simulink model "NowWereHere2018"  (R2018b)
settings: Solver=VariableStepAuto  StartTime=0.0  StopTime=120  MaxStep=10e-3  RelTol=1e-3
libraries: simulink x1, simulink_extras x1
settings Model: Creator=einarsu  LastModifiedBy=krist
settings OptimizationCC: LifeSpan=inf
settings SFSimCC: SimUseLocalCustomCode=off
settings RTWCC: RTWUseLocalCustomCode=off
settings CodeAppCC: StateflowObjectComments=on

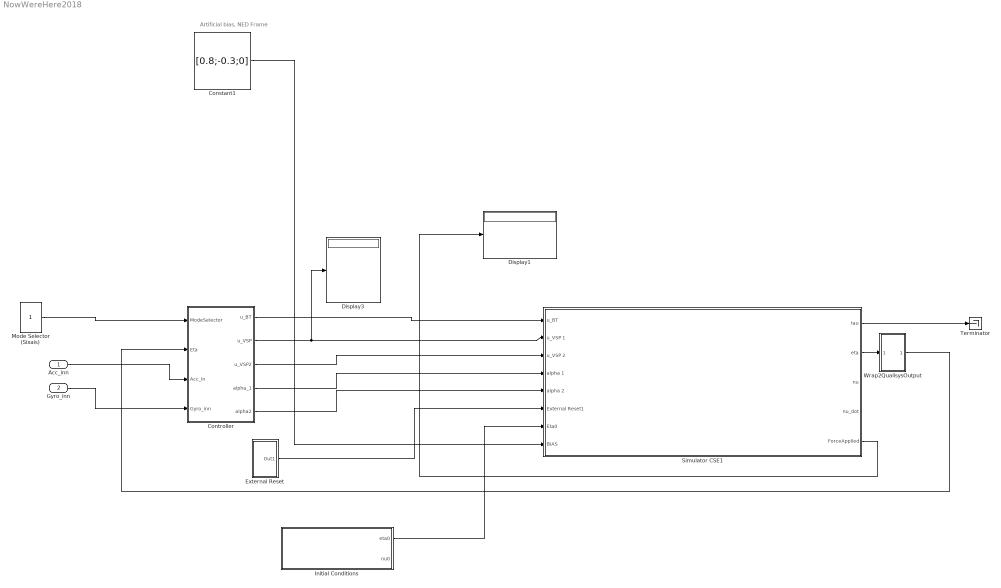
== system NowWereHere2018 ==
  note: Artificial bias, NED Frame
  Acc_inn : Inport
  Gyro_inn : Inport  Port=2
  Constant1 : Constant  Value=[0.8;-0.3;0]
  Controller : Subsystem
  Display1 : Display
  Display3 : Display
  External Reset : Subsystem
  "Initial Conditions " : Subsystem
  Mode Selector (Sixais) : Constant
  Simulator CSE1 : Subsystem
  Terminator : Terminator
  "Wrap2QualisysOutput " : Subsystem
  wires:
  Controller/1(u_BT) -> Simulator CSE1/1(u_BT)
  Controller/4(alpha_1) -> Simulator CSE1/4(alpha 1)
  Controller/2(u_VSP) -> Display3/1, Simulator CSE1/2(u_VSP 1)
  Controller/5(alpha2) -> Simulator CSE1/5(alpha 2)
  Controller/3("u_VSP2 ") -> Simulator CSE1/3(u_VSP 2)
  Simulator CSE1/1(tau) -> Terminator/1
  External Reset/1(Out1) -> Simulator CSE1/6(External Reset1)
  "Initial Conditions "/1(eta0) -> Simulator CSE1/7(Eta0)
  Mode Selector (Sixais)/1 -> Controller/1(ModeSelector)
  Simulator CSE1/2(eta) -> "Wrap2QualisysOutput "/1(In1)
  Acc_inn/1 -> Controller/3(Acc_in)
  Gyro_inn/1 -> Controller/4(Gyro_inn)
  Simulator CSE1/5(ForceApplied) -> Display1/1
  Constant1/1 -> Simulator CSE1/8(BIAS)
  "Wrap2QualisysOutput "/1(Out1) -> Controller/2(Eta)

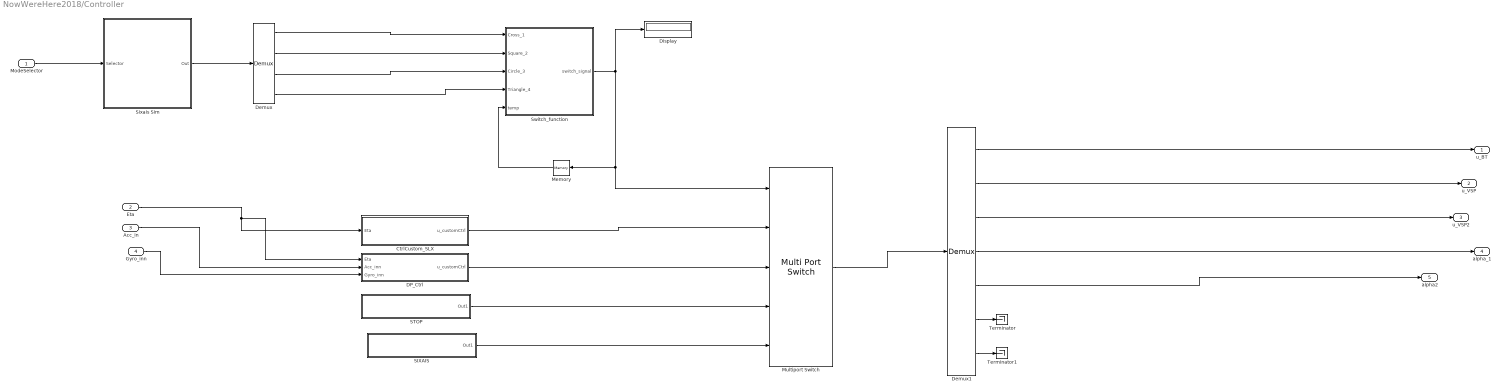
== system NowWereHere2018/Controller ==
  ModeSelector : Inport
  Eta : Inport  Port=2
  Acc_in : Inport  Port=3
  Gyro_inn : Inport  Port=4
  CtrlCustom_SLX : Subsystem
  DP_Ctrl : Subsystem
  Demux : Demux
  Demux1 : Demux  Outputs=7
  Display : Display
  Memory : Memory  InitialCondition=4
  Multiport Switch : MultiPortSwitch  Inputs=4
  SIXAIS : Subsystem
  STOP : Subsystem
  Sixais Sim : MATLAB Function  TreatAsAtomicUnit=on
  Switch_function : MATLAB Function  TreatAsAtomicUnit=on
  Terminator : Terminator
  Terminator1 : Terminator
  u_BT : Outport  VectorParamsAs1DForOutWhenUnconnected=off
  u_VSP : Outport  Port=2  VectorParamsAs1DForOutWhenUnconnected=off
  "u_VSP2 " : Outport  Port=3  VectorParamsAs1DForOutWhenUnconnected=off
  alpha_1 : Outport  Port=4  VectorParamsAs1DForOutWhenUnconnected=off
  alpha2 : Outport  Port=5  VectorParamsAs1DForOutWhenUnconnected=off
  wires:
  Switch_function/1(switch_signal) -> Memory/1, Multiport Switch/1, Display/1
  Memory/1 -> Switch_function/5(temp)
  CtrlCustom_SLX/1(u_customCtrl) -> Multiport Switch/2
  Demux/1 -> Switch_function/1(Cross_1)
  Demux/2 -> Switch_function/2(Square_2)
  Demux/3 -> Switch_function/3(Circle_3)
  Demux/4 -> Switch_function/4(Triangle_4)
  Sixais Sim/1(Out) -> Demux/1
  ModeSelector/1 -> Sixais Sim/1(Selector)
  DP_Ctrl/1(u_customCtrl) -> Multiport Switch/3
  STOP/1(Out1) -> Multiport Switch/4
  SIXAIS/1(Out1) -> Multiport Switch/5
  Eta/1 -> DP_Ctrl/1(Eta), CtrlCustom_SLX/1(Eta)
  Acc_in/1 -> DP_Ctrl/2(Acc_inn)
  Gyro_inn/1 -> DP_Ctrl/3(Gyro_inn)
  Multiport Switch/1 -> Demux1/1
  Demux1/1 -> u_BT/1
  Demux1/2 -> u_VSP/1
  Demux1/3 -> "u_VSP2 "/1
  Demux1/4 -> alpha_1/1
  Demux1/5 -> alpha2/1
  Demux1/6 -> Terminator/1
  Demux1/7 -> Terminator1/1

== system NowWereHere2018/External Reset ==
  note: Most relevant for Real-Time Simulations...
  Constant : Constant  Value=0
  Out1 : Outport  VectorParamsAs1DForOutWhenUnconnected=off
  wires:
  Constant/1 -> Out1/1

== system NowWereHere2018/Initial Conditions  ==
  Eta0 : Constant  Value=zeros(3,1)
  "V0 " : Constant  Value=zeros(3,1)
  eta0 : Outport  VectorParamsAs1DForOutWhenUnconnected=off
  nu0 : Outport  Port=2  VectorParamsAs1DForOutWhenUnconnected=off
  wires:
  "V0 "/1 -> nu0/1
  Eta0/1 -> eta0/1

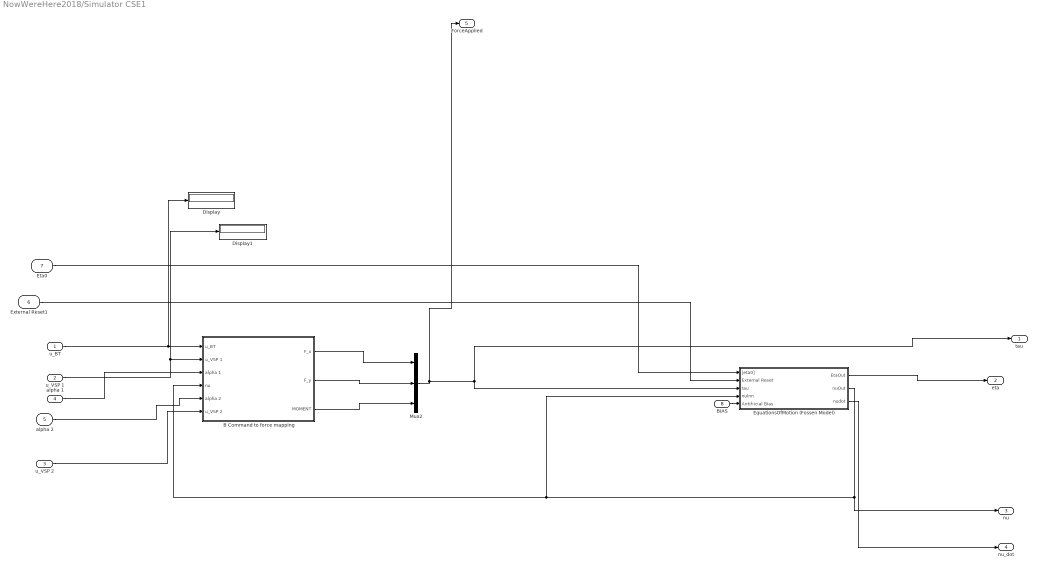
== system NowWereHere2018/Simulator CSE1 ==
  u_BT : Inport
  u_VSP 1 : Inport  Port=2
  u_VSP 2 : Inport  Port=3
  alpha 1 : Inport  Port=4
  alpha 2 : Inport  Port=5
  External Reset1 : Inport  Port=6
  Eta0 : Inport  Port=7
  BIAS : Inport  Port=8
  B Command to force mapping : Subsystem
  Display : Display
  Display1 : Display
  EquationsOfMotion (Fossen Model) : Subsystem
  Mux2 : Mux  Inputs=3
  tau : Outport  VectorParamsAs1DForOutWhenUnconnected=off
  eta : Outport  Port=2  VectorParamsAs1DForOutWhenUnconnected=off
  nu : Outport  Port=3  VectorParamsAs1DForOutWhenUnconnected=off
  nu_dot : Outport  Port=4  VectorParamsAs1DForOutWhenUnconnected=off
  ForceApplied : Outport  Port=5  VectorParamsAs1DForOutWhenUnconnected=off
  wires:
  alpha 2/1 -> B Command to force mapping/5(alpha 2)
  B Command to force mapping/2("F_y ") -> Mux2/2
  B Command to force mapping/1(F_x) -> Mux2/1
  u_VSP 1/1 -> B Command to force mapping/2(u_VSP 1), Display1/1
  alpha 1/1 -> B Command to force mapping/3(alpha 1)
  u_BT/1 -> B Command to force mapping/1(u_BT), Display/1
  u_VSP 2/1 -> B Command to force mapping/6(u_VSP 2)
  EquationsOfMotion (Fossen Model)/2(nuOut) -> B Command to force mapping/4(nu), EquationsOfMotion (Fossen Model)/4(nuInn), nu/1
  Eta0/1 -> EquationsOfMotion (Fossen Model)/1("[eta0] ")
  External Reset1/1 -> EquationsOfMotion (Fossen Model)/2(External Reset)
  Mux2/1 -> ForceApplied/1, EquationsOfMotion (Fossen Model)/3(tau), tau/1
  EquationsOfMotion (Fossen Model)/1(EtaOut) -> eta/1
  EquationsOfMotion (Fossen Model)/3(nudot) -> nu_dot/1
  B Command to force mapping/3("MOMENT ") -> Mux2/3
  BIAS/1 -> EquationsOfMotion (Fossen Model)/5(Aritifiicial BIas)

== system NowWereHere2018/Wrap2QualisysOutput  ==
  In1 : Inport
  Demux : Demux  Outputs=3
  Gain : Gain  Gain=1000
  Gain1 : Gain  Gain=1000
  Gain2 : Gain  Gain=180/pi
  Mux : Mux  Inputs=3
  Wrap2psi : MATLAB Function  TreatAsAtomicUnit=on
  Out1 : Outport  VectorParamsAs1DForOutWhenUnconnected=off
  wires:
  Mux/1 -> Out1/1
  In1/1 -> Demux/1
  Demux/3 -> Wrap2psi/1(u)
  Demux/1 -> Gain/1
  Demux/2 -> Gain1/1
  Gain/1 -> Mux/1
  Gain1/1 -> Mux/2
  Gain2/1 -> Mux/3
  Wrap2psi/1(yQualisus) -> Gain2/1

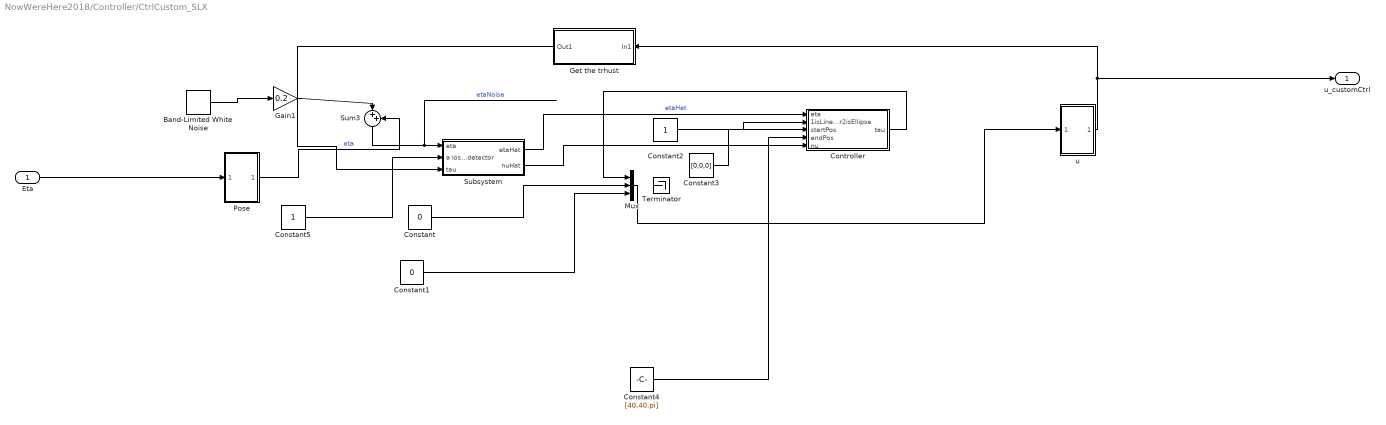
== system NowWereHere2018/Controller/CtrlCustom_SLX ==
  Eta : Inport
  Band-Limited White Noise : simulink/Sources/Band-Limited White Noise  Cov=[0.1]  Ts=0.1  seed=[23341]
  Constant : Constant  Value=0
  Constant1 : Constant  Value=0
  Constant2 : Constant
  Constant3 : Constant  Value=[0,0,0]
  Constant4 : Constant  Value=[40,40,pi]
  Constant5 : Constant
  Controller : Subsystem
  Gain1 : Gain  Gain=0.2
  Get the trhust : Subsystem
  Mux : Mux  Inputs=3
  Pose : Subsystem
  Subsystem : Subsystem
  Sum3 : Sum  Inputs=|++
  Terminator : Terminator
  u : Subsystem
  u_customCtrl : Outport  VectorParamsAs1DForOutWhenUnconnected=off
  wires:
  Eta/1 -> Pose/1(eta)
  Constant1/1 -> Mux/3
  Constant/1 -> Mux/2
  Pose/1(QTM) -> Sum3/2  "eta"
  Subsystem/1(etaHat) -> Controller/1(eta)  "etaHat"
  Constant5/1 -> Subsystem/2(a loss-of-signal detector)
  u/1(Out1) -> Get the trhust/1(In1), u_customCtrl/1
  Get the trhust/1(Out1) -> Subsystem/3(tau)
  Band-Limited White Noise/1 -> Gain1/1
  Gain1/1 -> Sum3/1
  Sum3/1 -> Subsystem/1(eta)  "etaNoise"
  Controller/1(tau) -> Mux/1
  Mux/1 -> u/1(In1)
  Constant2/1 -> Controller/2(1isLinear2isEllipse)
  Constant3/1 -> Controller/3(startPos)
  Constant4/1 -> Controller/4(endPos)
  Subsystem/2(nuHat) -> Controller/5(nu)

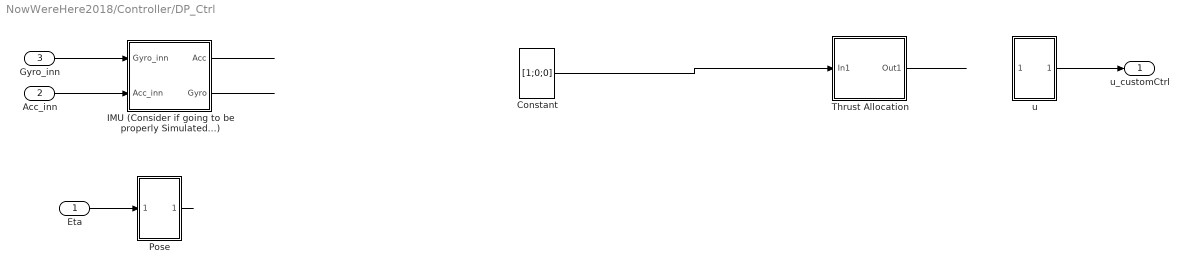
== system NowWereHere2018/Controller/DP_Ctrl ==
  Eta : Inport
  Acc_inn : Inport  Port=2
  Gyro_inn : Inport  Port=3
  Constant : Constant  Value=[1;0;0]
  IMU (Consider if going to be properly Simulated...) : Subsystem
  Pose : Subsystem
  "Thrust Allocation " : Subsystem
  u : Subsystem
  u_customCtrl : Outport  VectorParamsAs1DForOutWhenUnconnected=off
  wires:
  Pose/1(QTM) -> ?
  Gyro_inn/1 -> IMU (Consider if going to be properly Simulated...)/1(Gyro_inn)
  Acc_inn/1 -> IMU (Consider if going to be properly Simulated...)/2(Acc_inn)
  Eta/1 -> Pose/1(eta)
  u/1(Out1) -> u_customCtrl/1
  IMU (Consider if going to be properly Simulated...)/2(Gyro) -> ?
  IMU (Consider if going to be properly Simulated...)/1(Acc) -> ?
  Constant/1 -> "Thrust Allocation "/1(In1)
  "Thrust Allocation "/1(Out1) -> ?

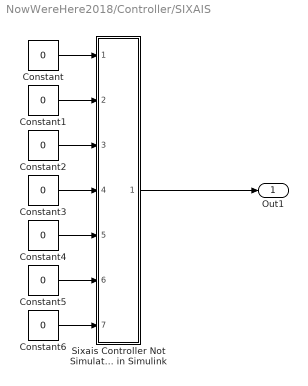
== system NowWereHere2018/Controller/SIXAIS ==
  Constant{,1..6} (7 alike) : Constant  Value=0
  Sixais Controller Not Simulated in Simulink : Subsystem
  Out1 : Outport  VectorParamsAs1DForOutWhenUnconnected=off
  wires:
  Constant/1 -> Sixais Controller Not Simulated in Simulink/1(In1)
  Constant1/1 -> Sixais Controller Not Simulated in Simulink/2(In2)
  Constant2/1 -> Sixais Controller Not Simulated in Simulink/3(In3)
  Constant3/1 -> Sixais Controller Not Simulated in Simulink/4(In4)
  Constant4/1 -> Sixais Controller Not Simulated in Simulink/5(In5)
  Constant5/1 -> Sixais Controller Not Simulated in Simulink/6(In6)
  Constant6/1 -> Sixais Controller Not Simulated in Simulink/7(In7)
  Sixais Controller Not Simulated in Simulink/1(Out1) -> Out1/1

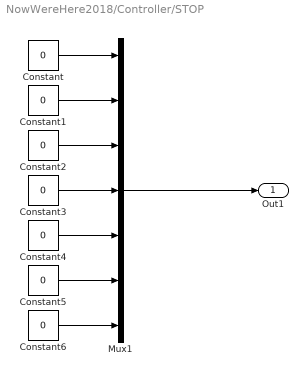
== system NowWereHere2018/Controller/STOP ==
  Constant{,1..6} (7 alike) : Constant  Value=0
  Mux1 : Mux  Inputs=7
  Out1 : Outport  VectorParamsAs1DForOutWhenUnconnected=off
  wires:
  Mux1/1 -> Out1/1
  Constant/1 -> Mux1/1
  Constant1/1 -> Mux1/2
  Constant2/1 -> Mux1/3
  Constant3/1 -> Mux1/4
  Constant4/1 -> Mux1/5
  Constant5/1 -> Mux1/6
  Constant6/1 -> Mux1/7

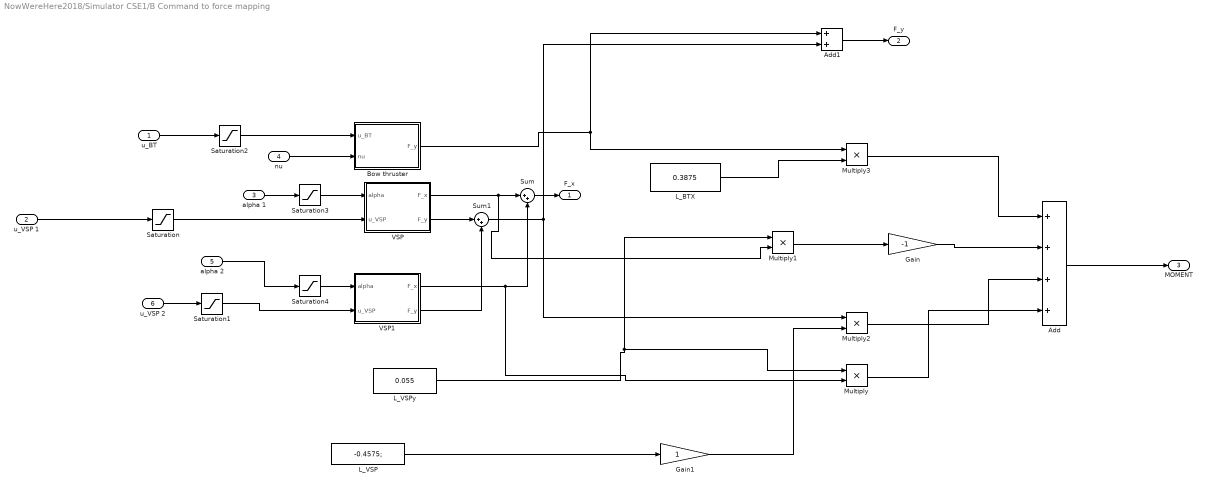
== system NowWereHere2018/Simulator CSE1/B Command to force mapping ==
  u_BT : Inport
  u_VSP 1 : Inport  Port=2
  alpha 1 : Inport  Port=3
  nu : Inport  Port=4
  alpha 2 : Inport  Port=5
  u_VSP 2 : Inport  Port=6
  Add : Sum  Inputs=++++
  Add1 : Sum
  Bow thruster : MATLAB Function  TreatAsAtomicUnit=on
  Gain : Gain  Gain=-1
  Gain1 : Gain
  L_BTX : Constant  Value=0.3875
  L_VSP : Constant  Value=-0.4575;
  L_VSPy : Constant  Value=0.055
  Multiply{,1..3} (4 alike) : Product
  Saturation : Saturate  UpperLimit=1  LowerLimit=0
  Saturation1 : Saturate  UpperLimit=1  LowerLimit=0
  Saturation2 : Saturate  UpperLimit=1  LowerLimit=-1
  Saturation3 : Saturate  UpperLimit=pi  LowerLimit=-pi
  Saturation4 : Saturate  UpperLimit=pi  LowerLimit=-pi
  Sum : Sum  Inputs=|++
  Sum1 : Sum  Inputs=|++
  VSP : MATLAB Function  TreatAsAtomicUnit=on
  VSP1 : MATLAB Function  TreatAsAtomicUnit=on
  F_x : Outport  VectorParamsAs1DForOutWhenUnconnected=off
  "F_y " : Outport  Port=2  VectorParamsAs1DForOutWhenUnconnected=off
  "MOMENT " : Outport  Port=3  VectorParamsAs1DForOutWhenUnconnected=off
  wires:
  alpha 1/1 -> Saturation3/1
  nu/1 -> Bow thruster/2(nu)
  Bow thruster/1(F_y) -> Add1/1, Multiply3/1
  VSP/2(F_y) -> Sum1/1
  Sum1/1 -> Add1/2, Multiply2/1
  VSP1/2(F_y) -> Sum1/2
  VSP1/1(F_x) -> Multiply/2, Sum/2
  VSP/1(F_x) -> Multiply1/2, Sum/1
  Sum/1 -> F_x/1
  alpha 2/1 -> Saturation4/1
  u_VSP 2/1 -> Saturation1/1
  L_VSP/1 -> Gain1/1
  L_BTX/1 -> Multiply3/2
  L_VSPy/1 -> Multiply/1, Multiply1/1
  Multiply3/1 -> Add/1
  Multiply1/1 -> Gain/1
  Multiply2/1 -> Add/3
  Multiply/1 -> Add/4
  Add/1 -> "MOMENT "/1
  Gain/1 -> Add/2
  Gain1/1 -> Multiply2/2
  Add1/1 -> "F_y "/1
  Saturation/1 -> VSP/2(u_VSP)
  Saturation1/1 -> VSP1/2(u_VSP)
  u_BT/1 -> Saturation2/1
  u_VSP 1/1 -> Saturation/1
  Saturation2/1 -> Bow thruster/1(u_BT)
  Saturation3/1 -> VSP/1(alpha)
  Saturation4/1 -> VSP1/1(alpha)

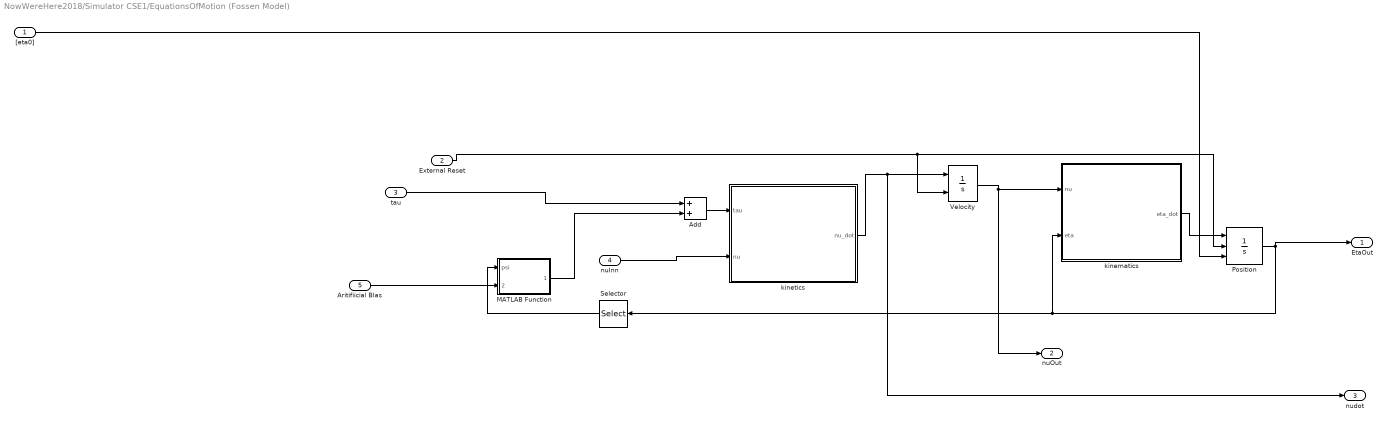
== system NowWereHere2018/Simulator CSE1/EquationsOfMotion (Fossen Model) ==
  "[eta0] " : Inport
  External Reset : Inport  Port=2
  tau : Inport  Port=3
  nuInn : Inport  Port=4
  Aritifiicial BIas : Inport  Port=5
  Add : Sum
  MATLAB Function : MATLAB Function  TreatAsAtomicUnit=on
  Position : Integrator  ExternalReset=either  InitialConditionSource=external  InitialCondition=[0 0 0]'
  Selector : Selector  InputPortWidth=3  IndexOptions=Index vector (dialog)  Indices=[3]  OutputSizes=1
  Velocity : Integrator  ExternalReset=either  InitialCondition=[0 0 0]'
  kinematics : MATLAB Function  TreatAsAtomicUnit=on
  kinetics : MATLAB Function  TreatAsAtomicUnit=on
  EtaOut : Outport  VectorParamsAs1DForOutWhenUnconnected=off
  nuOut : Outport  Port=2  VectorParamsAs1DForOutWhenUnconnected=off
  nudot : Outport  Port=3  VectorParamsAs1DForOutWhenUnconnected=off
  wires:
  tau/1 -> Add/1
  Position/1 -> Selector/1, kinematics/2(eta), EtaOut/1
  "[eta0] "/1 -> Position/3
  nuInn/1 -> kinetics/2(nu)
  kinematics/1(eta_dot) -> Position/1
  Velocity/1 -> nuOut/1, kinematics/1(nu)
  kinetics/1(nu_dot) -> nudot/1, Velocity/1
  External Reset/1 -> Velocity/2, Position/2
  Add/1 -> kinetics/1(tau)
  Aritifiicial BIas/1 -> MATLAB Function/2(NedVector)
  Selector/1 -> MATLAB Function/1(psi)
  MATLAB Function/1(BodyVector) -> Add/2

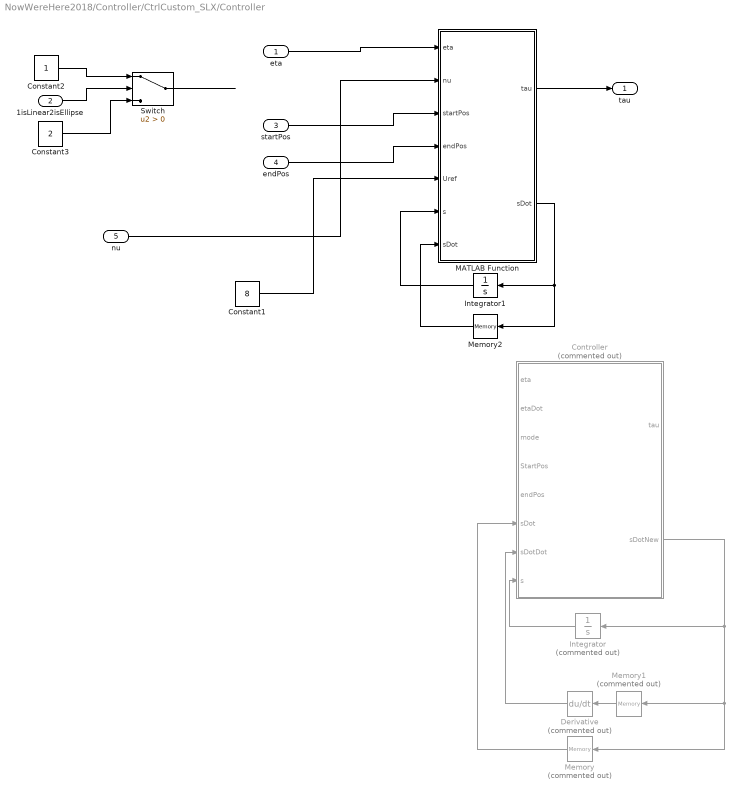
== system NowWereHere2018/Controller/CtrlCustom_SLX/Controller ==
  eta : Inport
  1isLinear2isEllipse : Inport  Port=2
  startPos : Inport  Port=3
  endPos : Inport  Port=4
  nu : Inport  Port=5  PortDimensions=3
  Constant1 : Constant  Value=8
  Constant2 : Constant
  Constant3 : Constant  Value=2
  Controller : MATLAB Function  Commented=on  TreatAsAtomicUnit=on
  Derivative : Derivative  Commented=on
  Integrator : Integrator  Commented=on
  Integrator1 : Integrator
  MATLAB Function : MATLAB Function  TreatAsAtomicUnit=on
  Memory : Memory  Commented=on
  Memory1 : Memory  Commented=on
  Memory2 : Memory
  Switch : Switch  Criteria=u2 > Threshold
  tau : Outport
  wires:
  MATLAB Function/1(tau) -> tau/1
  Integrator/1 -> Controller/8(s)
  eta/1 -> MATLAB Function/1(eta)
  Switch/1 -> ?
  Constant3/1 -> Switch/3
  1isLinear2isEllipse/1 -> Switch/2
  Constant2/1 -> Switch/1
  Controller/2(sDotNew) -> Memory/1, Memory1/1, Integrator/1
  Memory/1 -> Controller/6(sDot)
  endPos/1 -> MATLAB Function/4(endPos)
  startPos/1 -> MATLAB Function/3(startPos)
  Derivative/1 -> Controller/7(sDotDot)
  nu/1 -> MATLAB Function/2(nu)
  Memory1/1 -> Derivative/1
  MATLAB Function/2(sDot) -> Integrator1/1, Memory2/1
  Memory2/1 -> MATLAB Function/7("sDot ")
  Integrator1/1 -> MATLAB Function/6(s)
  Constant1/1 -> MATLAB Function/5(Uref)

== system NowWereHere2018/Controller/CtrlCustom_SLX/Get the trhust ==
  In1 : Inport
  Demux : Demux  Outputs=7
  Mux : Mux  Inputs=3
  Terminator{,1..3} (4 alike) : Terminator
  Out1 : Outport  VectorParamsAs1DForOutWhenUnconnected=off
  wires:
  In1/1 -> Demux/1
  Demux/3 -> Mux/3
  Demux/1 -> Mux/1
  Demux/2 -> Mux/2
  Demux/7 -> Terminator/1
  Demux/6 -> Terminator3/1
  Demux/5 -> Terminator2/1
  Demux/4 -> Terminator1/1
  Mux/1 -> Out1/1

== system NowWereHere2018/Controller/CtrlCustom_SLX/Pose ==
  eta : Inport
  Degrees to Radians : simulink_extras/Transformations/Degrees to Radians
  Demux : Demux  Outputs=3
  Gain : Gain  Gain=0.001000
  Gain1 : Gain  Gain=0.001000
  MATLAB Function : MATLAB Function  TreatAsAtomicUnit=on
  Memory : Memory
  Mux : Mux  Inputs=3
  QTM : Outport  PortDimensions=3  VectorParamsAs1DForOutWhenUnconnected=off
  wires:
  Demux/2 -> Gain/1  "y_m"
  Demux/3 -> Degrees to Radians/1  "psi_m"
  Demux/1 -> Gain1/1  "x_m"
  Mux/1 -> QTM/1
  eta/1 -> Demux/1
  Gain/1 -> Mux/2
  Gain1/1 -> Mux/1
  Degrees to Radians/1 -> MATLAB Function/1(newAng)
  MATLAB Function/1(retAng) -> Memory/1, Mux/3  "eta"
  Memory/1 -> MATLAB Function/2(oldAng)

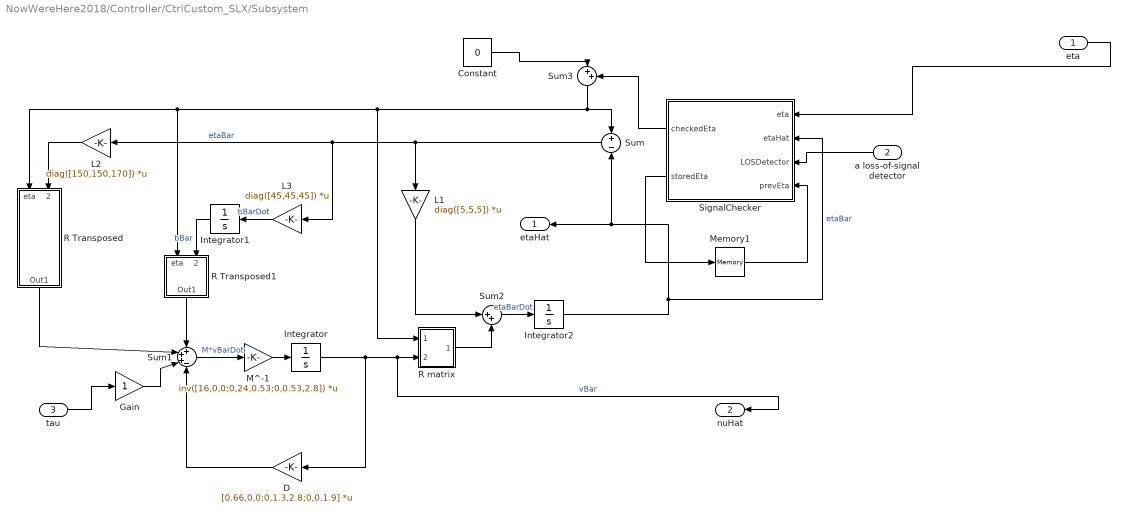
== system NowWereHere2018/Controller/CtrlCustom_SLX/Subsystem ==
  eta : Inport
  a loss-of-signal detector : Inport  Port=2
  tau : Inport  Port=3
  Constant : Constant  Value=0
  D : Gain  Gain=[0.66,0,0;0,1.3,2.8;0,0,1.9]  Multiplication=Matrix(K*u)
  Gain : Gain
  Integrator : Integrator
  Integrator1 : Integrator
  Integrator2 : Integrator
  L1 : Gain  Gain=diag([5,5,5])  Multiplication=Matrix(K*u)
  L2 : Gain  Gain=diag([150,150,170])  Multiplication=Matrix(K*u)
  L3 : Gain  Gain=diag([45,45,45])  Multiplication=Matrix(K*u)
  M^-1 : Gain  Gain=inv([16,0,0;0,24,0.53;0,0.53,2.8])  Multiplication=Matrix(K*u)
  Memory1 : Memory  InitialCondition=[0,0,0; 0,0,0; 0,0,0]
  R Transposed : Subsystem
  R Transposed1 : Subsystem
  "R matrix " : Subsystem
  SignalChecker : MATLAB Function  TreatAsAtomicUnit=on
  Sum : Sum  Inputs=+|-
  Sum1 : Sum  Inputs=+++-
  Sum2 : Sum  Inputs=|++
  Sum3 : Sum  Inputs=|++
  etaHat : Outport  VectorParamsAs1DForOutWhenUnconnected=off
  nuHat : Outport  Port=2  PortDimensions=3  VectorParamsAs1DForOutWhenUnconnected=off
  wires:
  Sum/1 -> L1/1, L3/1, L2/1  "etaBar"
  M^-1/1 -> Integrator/1
  Sum1/1 -> M^-1/1  "M*vBarDot"
  D/1 -> Sum1/4
  R Transposed1/1(Out1) -> Sum1/1
  Integrator1/1 -> R Transposed1/2(etaBar)  "bBar"
  L3/1 -> Integrator1/1  "bBarDot"
  Integrator/1 -> D/1, nuHat/1, "R matrix "/2(etaBar)  "vBar"
  "R matrix "/1(Out1) -> Sum2/2
  L1/1 -> Sum2/1
  Sum2/1 -> Integrator2/1  "etaBarDot"
  R Transposed/1(Out1) -> Sum1/2
  a loss-of-signal detector/1 -> SignalChecker/3(LOSDetector)
  Memory1/1 -> SignalChecker/4(prevEta)
  SignalChecker/2(storedEta) -> Memory1/1
  Sum3/1 -> Sum/1, R Transposed1/1(eta), R Transposed/1(eta), "R matrix "/1(eta)
  SignalChecker/1(checkedEta) -> Sum3/2
  Constant/1 -> Sum3/1
  L2/1 -> R Transposed/2(etaBar)
  tau/1 -> Gain/1
  Gain/1 -> Sum1/3
  eta/1 -> SignalChecker/1(eta)
  Integrator2/1 -> Sum/2, etaHat/1, SignalChecker/2(etaHat)  "etaBar"

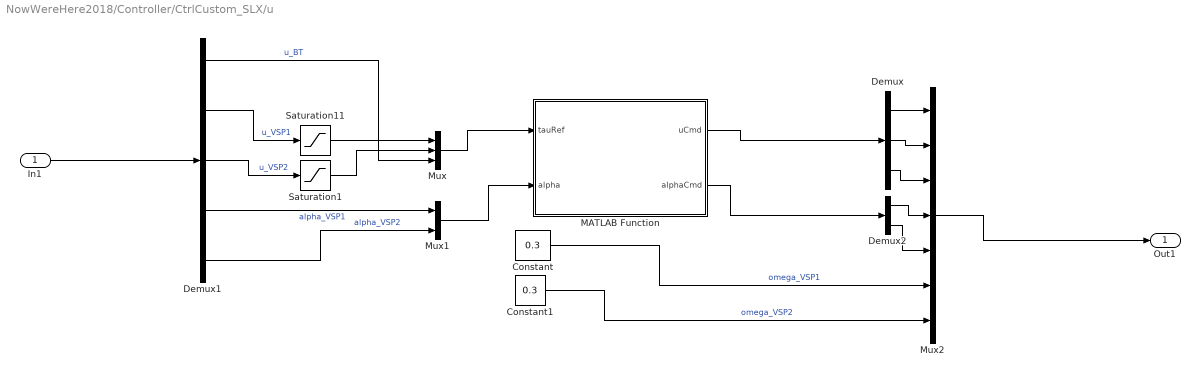
== system NowWereHere2018/Controller/CtrlCustom_SLX/u ==
  In1 : Inport
  Constant : Constant  Value=0.3
  Constant1 : Constant  Value=0.3
  Demux : Demux  Outputs=3
  Demux1 : Demux  Outputs=5
  Demux2 : Demux  Outputs=2
  MATLAB Function : MATLAB Function  TreatAsAtomicUnit=on
  Mux : Mux  Inputs=3
  Mux1 : Mux  Inputs=2
  Mux2 : Mux  Inputs=7
  Saturation1 : Saturate  UpperLimit=1  LowerLimit=0
  Saturation11 : Saturate  UpperLimit=1  LowerLimit=0
  Out1 : Outport  VectorParamsAs1DForOutWhenUnconnected=off
  wires:
  In1/1 -> Demux1/1
  Demux1/1 -> Mux/3  "u_BT"
  Demux1/2 -> Saturation11/1  "u_VSP1"
  Demux1/3 -> Saturation1/1  "u_VSP2"
  Demux1/4 -> Mux1/1  "alpha_VSP1"
  Demux1/5 -> Mux1/2  "alpha_VSP2"
  Constant/1 -> Mux2/6  "omega_VSP1"
  Constant1/1 -> Mux2/7  "omega_VSP2"
  Saturation11/1 -> Mux/1
  Saturation1/1 -> Mux/2
  Mux/1 -> MATLAB Function/1(tauRef)
  Mux1/1 -> MATLAB Function/2(alpha)
  MATLAB Function/1(uCmd) -> Demux/1
  MATLAB Function/2(alphaCmd) -> Demux2/1
  Demux/1 -> Mux2/1
  Demux/2 -> Mux2/2
  Demux/3 -> Mux2/3
  Demux2/2 -> Mux2/5
  Demux2/1 -> Mux2/4
  Mux2/1 -> Out1/1

== system NowWereHere2018/Controller/DP_Ctrl/IMU (Consider if going to be properly Simulated...) ==
  Gyro_inn : Inport
  Acc_inn : Inport  Port=2
  Demux : Demux  Outputs=3
  Demux1 : Demux  Outputs=3
  Mux : Mux  Inputs=3
  Mux2 : Mux  Inputs=3
  Acc : Outport  VectorParamsAs1DForOutWhenUnconnected=off
  Gyro : Outport  Port=2  VectorParamsAs1DForOutWhenUnconnected=off
  wires:
  Acc_inn/1 -> Demux1/1
  Gyro_inn/1 -> Demux/1
  Demux/1 -> Mux2/1
  Demux/2 -> Mux2/2
  Demux/3 -> Mux2/3
  Demux1/2 -> Mux/2
  Demux1/3 -> Mux/3
  Mux2/1 -> Gyro/1
  Demux1/1 -> Mux/1
  Mux/1 -> Acc/1

== system NowWereHere2018/Controller/DP_Ctrl/Pose ==
  eta : Inport
  Demux : Demux  Outputs=3
  Mux : Mux  Inputs=3
  QTM : Outport  VectorParamsAs1DForOutWhenUnconnected=off
  wires:
  eta/1 -> Demux/1
  Mux/1 -> QTM/1
  Demux/1 -> Mux/1  "x_m"
  Demux/3 -> Mux/3  "psi_m"
  Demux/2 -> Mux/2  "y_m"

== system NowWereHere2018/Controller/DP_Ctrl/Thrust Allocation  ==
  In1 : Inport
  THALOC (u->tau) : MATLAB Function  TreatAsAtomicUnit=on
  Out1 : Outport  VectorParamsAs1DForOutWhenUnconnected=off
  wires:
  In1/1 -> THALOC (u->tau)/1(u)
  THALOC (u->tau)/1(y) -> Out1/1

== system NowWereHere2018/Controller/DP_Ctrl/u ==
  In1 : Inport
  Demux1 : Demux  Outputs=7
  Mux : Mux  Inputs=7
  Out1 : Outport  VectorParamsAs1DForOutWhenUnconnected=off
  wires:
  Mux/1 -> Out1/1
  Demux1/7 -> Mux/7  "omega_VSP2"
  Demux1/6 -> Mux/6  "omega_VSP1"
  Demux1/5 -> Mux/5  "alpha_VSP2"
  Demux1/4 -> Mux/4  "alpha_VSP1"
  Demux1/3 -> Mux/3  "u_VSP2"
  Demux1/2 -> Mux/2  "u_VSP1"
  Demux1/1 -> Mux/1  "u_BT"
  In1/1 -> Demux1/1

== system NowWereHere2018/Controller/SIXAIS/Sixais Controller Not Simulated in Simulink ==
  In1 : Inport
  In2 : Inport  Port=2
  In3 : Inport  Port=3
  In4 : Inport  Port=4
  In5 : Inport  Port=5
  In6 : Inport  Port=6
  In7 : Inport  Port=7
  Mux1 : Mux  Inputs=7
  Out1 : Outport  VectorParamsAs1DForOutWhenUnconnected=off
  wires:
  In4/1 -> Mux1/4
  In5/1 -> Mux1/5
  In6/1 -> Mux1/6
  In3/1 -> Mux1/3
  In1/1 -> Mux1/1
  In2/1 -> Mux1/2
  Mux1/1 -> Out1/1
  In7/1 -> Mux1/7

== system NowWereHere2018/Controller/CtrlCustom_SLX/Subsystem/R Transposed ==
  eta : Inport
  etaBar : Inport  Port=2
  Mux : Mux  Inputs=2
  Mux1 : Mux  Inputs=3
  Row1 : Fcn  Expr=cos(u(1))*u(2)+sin(u(1))*u(3)
  Row2 : Fcn  Expr=-sin(u(1))*u(2)+cos(u(1))*u(3)
  Row3 : Fcn  Expr=u(4)
  yaw angle : Fcn  Expr=u(3)
  Out1 : Outport  VectorParamsAs1DForOutWhenUnconnected=off
  wires:
  Mux1/1 -> Out1/1
  etaBar/1 -> Mux/2
  Mux/1 -> Row3/1, Row2/1, Row1/1
  Row1/1 -> Mux1/1
  Row3/1 -> Mux1/3
  Row2/1 -> Mux1/2
  eta/1 -> yaw angle/1
  yaw angle/1 -> Mux/1  "psi"

== system NowWereHere2018/Controller/CtrlCustom_SLX/Subsystem/R Transposed1 ==
  eta : Inport
  etaBar : Inport  Port=2
  Mux : Mux  Inputs=2
  Mux1 : Mux  Inputs=3
  Row1 : Fcn  Expr=cos(u(1))*u(2)+sin(u(1))*u(3)
  Row2 : Fcn  Expr=-sin(u(1))*u(2)+cos(u(1))*u(3)
  Row3 : Fcn  Expr=u(4)
  yaw angle : Fcn  Expr=u(3)
  Out1 : Outport  VectorParamsAs1DForOutWhenUnconnected=off
  wires:
  Mux1/1 -> Out1/1
  etaBar/1 -> Mux/2
  Mux/1 -> Row3/1, Row2/1, Row1/1
  Row1/1 -> Mux1/1
  Row3/1 -> Mux1/3
  Row2/1 -> Mux1/2
  eta/1 -> yaw angle/1
  yaw angle/1 -> Mux/1  "psi"

== system NowWereHere2018/Controller/CtrlCustom_SLX/Subsystem/R matrix  ==
  eta : Inport
  etaBar : Inport  Port=2
  Mux : Mux  Inputs=2
  Mux1 : Mux  Inputs=3
  Row1 : Fcn  Expr=cos(u(1))*u(2)-sin(u(1))*u(3)
  Row2 : Fcn  Expr=sin(u(1))*u(2)+cos(u(1))*u(3)
  Row3 : Fcn  Expr=u(4)
  yaw angle : Fcn  Expr=u(3)
  Out1 : Outport  VectorParamsAs1DForOutWhenUnconnected=off
  wires:
  Mux1/1 -> Out1/1
  etaBar/1 -> Mux/2
  Mux/1 -> Row3/1, Row2/1, Row1/1
  Row1/1 -> Mux1/1
  Row3/1 -> Mux1/3
  Row2/1 -> Mux1/2
  eta/1 -> yaw angle/1
  yaw angle/1 -> Mux/1  "psi"

== matlab function NowWereHere2018/Simulator CSE1/EquationsOfMotion (Fossen Model)/kinematics ==
  data: nu input; eta_dot output; eta input
function eta_dot = CSE1_eta_dot(nu,eta)

psi = eta(3);

J = [cos(psi) -sin(psi) 0
     sin(psi) cos(psi)  0
     0        0         1];

eta_dot = J*nu;

== matlab function NowWereHere2018/Simulator CSE1/EquationsOfMotion (Fossen Model)/kinetics ==
  data: tau input; nu_dot output; nu input
function nu_dot = CSE1_nu_dot(tau,nu)

u   = nu(1);
v   = nu(2);
r   = nu(3);

tau = [tau(1);tau(2);tau(3)];
%% MATRICES 
%changed m from 14.79 to 14.11

m    = 14.11;   I_z  =  1.7600;   x_g = 0.0375;       % x_g  =  0.0460; % Table B.1

%% Added mass
%changed Y_vd from -1.0 to -10.0
X_ud  =     -2.0;											% Table B.1
					Y_vd =      -10.0;	N_vd =    -0.0;		% Table B.1
					Y_rd =      -0.0;	N_rd =    -1.0;		% Table B.1

%% Total mass matrix
m_11 = m-X_ud;
m_22 = m-Y_vd;
m_23 = m*x_g-Y_rd;
m_32 = m*x_g-N_vd; % noted as Y_rd in handbook, but same value
m_33 = I_z-N_rd;

M    = [m_11 0    0
        0    m_22 m_23
        0    m_32 m_33];
	
%% Damping coefficients
% Comments at the end of the lines indicate the old values used.
X_u		= -0.6555;		X_v		= 0;
X_uu 	= 0.3545;		X_vv	= -2.443;
X_uuu 	= -3.787;		X_vvv	= 0;

						Y_v		= -1.33; 			Y_r		= -7.250; % Y_r
						Y_vv	= -2.776;			Y_rr	= -3.450; % Y_rr
						Y_vvv	= -64.91;			Y_rrr	= 0;
						
						Y_rv	= -0.805;			Y_vr	= -0.845; % Y_rv, Y_vr

						N_v		= 0;				N_r		= -1.900; % N_r
						N_vv	= -0.2088;			N_rr	= -0.750; % N_rr
						N_vvv	= 0;				N_rrr	= 0;
						
						N_rv	= 0.130;			N_vr	= 0.080; % N_rv, N_vr

%% Correolis matrix
c_13 = -(m-Y_vd)*v-(m*x_g-Y_rd)*r;
c_23 = (m-X_ud)*u;
C    = [0     0     c_13
        0     0     c_23
        -c_13 -c_23 0   ];

%% Assembly of the damping matrix
%should be abs(u), abs(v) some places, only positive values? 

d_11 = -X_u - X_uu*u - X_uuu*u^2;
d_22 = -Y_v - Y_vv*v - Y_vvv*v^2 - Y_rv*abs(r);
d_33 = -N_r - N_rr*abs(r) - N_rrr*r^2 - N_vr*abs(v); % using abs(r)

d_12 = -X_v - X_vv*v - X_vvv*v^2;
d_23 = -Y_r - Y_rr*abs(r) - Y_rrr*r^2 - Y_vr*abs(v);
d_32 = -N_v - N_vv*v - N_vvv*v^2 - N_rv*abs(r);

%D    = [d_11 d_12 0      vet ikke hvorfor d_12 er her
%        0    d_22 d_23
%        0    d_32 d_33];
D    = [d_11 0 0
        0    d_22 d_23
        0    d_32 d_33];


%% CALCULATION
nu_dot = M\(tau-(C+D)*nu);

== matlab function NowWereHere2018/Simulator CSE1/EquationsOfMotion (Fossen Model)/MATLAB Function ==
  data: psi input; BodyVector output; NedVector input
function BodyVector = fcn(psi,NedVector)
R=[cos(psi) sin(psi) 0; -sin(psi) cos(psi) 0;0 0 1];
BodyVector=R*NedVector;
end

== matlab function NowWereHere2018/Wrap2QualisysOutput /Wrap2psi ==
  data: u input; yQualisus output
function yQualisus = fcn(u)
y=sin(u)
x=cos(u)
yQualisus=atan2(y,x);
end

== matlab function NowWereHere2018/Controller/CtrlCustom_SLX/u/MATLAB Function ==
  data: tauRef input; uCmd output; alpha input; alphaCmd output
function [uCmd,alphaCmd]=ImplementingBetaFcnInSimulink(tauRef,alpha)
lx=0.055;
ly=0.4574;
K1 = 1.03;
K2 = K1;
K3 = 2.629;


K = diag([K1, K2, K3]);

Balpha=[cos(alpha(1)),cos(alpha(2)),0;sin(alpha(1)),sin(alpha(2)),1;-lx*cos(alpha(1))-lx*sin(alpha(1)),-ly*cos(alpha(2))-lx*sin(alpha(2)),lx];

uStar=pinv(Balpha*K)*tauRef;

Thrusters=2;
BowThrusters=1;

%test values
alphaCmd=alpha;
uCmd=uStar(:,1);
for i=1:Thrusters
    if uStar(i)<0
        uCmd(i)=-(uStar(i));
        if alpha(i)<0
            alphaCmd(i)=alpha(i)+pi;
        else
            alphaCmd(i)=alpha(i)-pi;
        end
    end
end
for i=Thrusters+1:BowThrusters
    uCmd(i)=uStar(i);
    
    
    
end
end

== matlab function NowWereHere2018/Controller/CtrlCustom_SLX/Subsystem/SignalChecker ==
  data: eta input; checkedEta output; etaHat input; LOSDetector input; prevEta input; storedEta output
function [checkedEta,storedEta]= fcn(eta,etaHat,LOSDetector,prevEta)



if LOSDetector
    deadSignal=true;
    for i=1:3
        if eta~=prevEta(i)
            deadSignal=false;
            break
        end
    end
    if deadSignal
        changeInEta = - prevEta(:,1) + prevEta(:,2);
        checkedEta = changeInEta(:,1) + prevEta(:,1);
    else
        checkedEta=eta;
    end
else
    changeInEta = prevEta(:,1) - prevEta(:,2);
    checkedEta = changeInEta(:,1) + prevEta(:,1);
end
storedEta=circshift(prevEta,1,2);
storedEta(:,1)=checkedEta;
end

== matlab function NowWereHere2018/Controller/CtrlCustom_SLX/Pose/MATLAB Function ==
  data: newAng input; retAng output; oldAng input
function retAng = fcn(newAng,oldAng)

retAng=oldAng+angdiff(oldAng,newAng);
end

== matlab function NowWereHere2018/Controller/Switch_function ==
  data: Cross_1 input; switch_signal output; Square_2 input; Circle_3 input; Triangle_4 input; temp input
%% Function that takes in impulse button sigals [0,1] and sends out a 
% different signal depentent pn which button has been pressed

function switch_signal = fcn(Cross_1,Square_2,Circle_3,Triangle_4,temp)
%#codegen
persistent signal;

signal = temp;

if Cross_1 ~= 0
    signal = 1;
end

if Square_2 ~= 0
    signal = 2;
end

if Circle_3 ~= 0
    signal = 3;
end
    
if Triangle_4 ~= 0
    signal = 4; 
end

switch_signal = signal;

== matlab function NowWereHere2018/Controller/Sixais Sim ==
  data: Selector input; Out output
%% Function that takes in impulse button sigals [0,1] and sends out a 
% different signal depentent pn which button has been pressed

function Out = fcn(Selector)
%#codegen
if Selector==1
    Out=[1 0 0 0];
elseif Selector==2
        Out=[0 1 0 0];
elseif Selector==4
        Out=[0 0 0 1];
else 
        Out=[0 0 1 0];

end

== matlab function NowWereHere2018/Controller/DP_Ctrl/Thrust Allocation /THALOC (u->tau) ==
  data: u input; y output
function y = fcn(u)

y = u;

== matlab function NowWereHere2018/Controller/CtrlCustom_SLX/Controller/MATLAB Function ==
  data: eta input; tau output; nu input; startPos input; endPos input; Uref input; s input; sDot input; sDot output
function [tau,sDot] = fcn2(eta,nu,startPos,endPos,Uref,s,sDot)
R=[cos(eta(3)),-sin(eta(3)),0;
    sin(eta(3)),cos(eta(3)),0;
0,0,1];
Rt=transpose(R);
S=[0,-nu(3),0;
    nu(3),0,0;
    0,0,0];
St=transpose(S);
M=[16,0,0;0,24,0.53;0,0.53,2.8];
D=[0.66,0,0;0,1.3,2.8;0,0,1.9];
Kv=diag([1;1;1]);
Kp=diag([1;1;1]);

%straight line path
etaD=[s*endPos(1)+(1-s)*startPos(1);
    s*endPos(2)+(1-s)*startPos(2);
    atan((endPos(2)-startPos(2))/(endPos(1)-endPos(1)))];

etaDs=[endPos(1)-startPos(1);
    endPos(2)-startPos(2);
    0];
etaDss=zeros(3,1);


Us=Uref/norm(etaDs);

Uss=-Uref*etaDs(1)/(etaDs(1)^2+etaDs(2)^2)^(3/2)*etaDss(1) + ...
    -Uref*etaDs(2)/(etaDs(1)^2+etaDs(2)^2)^(3/2)*etaDss(2);

mu=1;

z1=Rt*(eta-etaD);

V1s=-transpose(z1)*Rt*etaDs;

alpha1=-Kp*z1 +Rt*etaDs*Us;

z1Dot=-S*z1 + nu - Rt*etaDs*(Us-mu/norm(etaDs)*V1s);

sigma1=St*Rt*etaDs*Us + Rt*sDot*(etaDss*Us+etaDs*Uss);

alpha1Dot=-Kp*z1Dot+sigma1;

z2=nu-alpha1;

tau=D*alpha1+M*alpha1Dot-Kv*z2;
sDot=(Us-(mu/norm(etaDs))*V1s)';
end

== matlab function NowWereHere2018/Simulator CSE1/B Command to force mapping/Bow thruster ==
  data: u_BT input; F_y output; nu input
function F_y = fcn(u_BT,nu)
%#codegen
u = nu(1);
% Thruster characteristics
if u_BT >0
    u_BT=u_BT+ 0.059;
    a =        -548;
    b =       0.193;
    c =       548.2;
    d =      0.1992;
    y0 = -(a*exp(b*-u_BT) + c*exp(d*-u_BT));
elseif u_BT < 0
    u_BT=u_BT- 0.059;
    a =        -548;
    b =       0.193;
    c =       548.2;
    d =      0.1992;
    y0 = a*exp(b*u_BT) + c*exp(d*u_BT);
else
    y0 = 0;
end
% Thruster losses due to forward speed
a0 =      0.7561;
a1 =      0.3075;
b1 =      -10.22;
c1 =       2.947;
F_y = y0*(a0 + a1*atan(b1*u +c1))/1.1385;
F_y=F_y*2.62/2.7629;


%2019 changes- Some add-hock changes, because it did not make sense previously.

== matlab function NowWereHere2018/Simulator CSE1/B Command to force mapping/VSP ==
  data: alpha input; F_x output; u_VSP input; F_y output
function [ F_x , F_y ] = fcn(alpha,u_VSP)
%#codegen
% Calculating the force in x-direction
a1 =       1.107  ;
b1 =       1.001  ;
c1 =       1.564  ;
a2 =      0.3471 ;
b2 =      0.1397 ;
c2 =      -1.599  ;
a3 =      0.1558 ;
b3 =       1.993  ;
c3 =       1.886  ;
a4 =      0.1599 ;
b4 =       0.218  ;
c4 =       1.513  ;
a5 =     0.08237 ;
b5 =       2.986  ;
c5 =      -1.601  ;
a6 =     0.04641 ;
b6 =       3.964  ;
c6 =       1.738  ;
F_x =   u_VSP*( a1*sin(b1*alpha+c1) + ...
                a2*sin(b2*alpha+c2) + ...
                a3*sin(b3*alpha+c3) + ...
                a4*sin(b4*alpha+c4) + ...
                a5*sin(b5*alpha+c5) + ...
                a6*sin(b6*alpha+c6) );
% Calculating the force in y-direction
a1 =      0.7936 ;
b1 =       1.001  ;
c1 =     0.01605;
a2 =      0.2112 ;
b2 =       1.997  ;
c2 =     0.03229;
a3 =     0.07608;
b3 =       2.991  ;
c3 =       2.986  ;
a4 =     0.04817;
b4 =       3.999  ;
c4 =     -0.8668 ;
a5 =     0.01757;
b5 =       4.904  ;
c5 =      -2.622 ;
a6 =    -0.02089;
b6 =       5.068  ;
c6 =      0.2548 ;
F_y =   u_VSP*( a1*sin(b1*alpha+c1) + ...
                a2*sin(b2*alpha+c2) + ...
                a3*sin(b3*alpha+c3) + ...
                a4*sin(b4*alpha+c4) + ...
                a5*sin(b5*alpha+c5) + ...
                a6*sin(b6*alpha+c6));

== matlab function NowWereHere2018/Simulator CSE1/B Command to force mapping/VSP1 ==
  data: alpha input; F_x output; u_VSP input; F_y output
function [ F_x , F_y ] = fcn(alpha,u_VSP)
%#codegen
% Calculating the force in x-direction
a1 =       1.107  ;
b1 =       1.001  ;
c1 =       1.564  ;
a2 =      0.3471 ;
b2 =      0.1397 ;
c2 =      -1.599  ;
a3 =      0.1558 ;
b3 =       1.993  ;
c3 =       1.886  ;
a4 =      0.1599 ;
b4 =       0.218  ;
c4 =       1.513  ;
a5 =     0.08237 ;
b5 =       2.986  ;
c5 =      -1.601  ;
a6 =     0.04641 ;
b6 =       3.964  ;
c6 =       1.738  ;
F_x =   u_VSP*( a1*sin(b1*alpha+c1) + ...
                a2*sin(b2*alpha+c2) + ...
                a3*sin(b3*alpha+c3) + ...
                a4*sin(b4*alpha+c4) + ...
                a5*sin(b5*alpha+c5) + ...
                a6*sin(b6*alpha+c6) );
% Calculating the force in y-direction
a1 =      0.7936 ;
b1 =       1.001  ;
c1 =     0.01605;
a2 =      0.2112 ;
b2 =       1.997  ;
c2 =     0.03229;
a3 =     0.07608;
b3 =       2.991  ;
c3 =       2.986  ;
a4 =     0.04817;
b4 =       3.999  ;
c4 =     -0.8668 ;
a5 =     0.01757;
b5 =       4.904  ;
c5 =      -2.622 ;
a6 =    -0.02089;
b6 =       5.068  ;
c6 =      0.2548 ;
F_y =   u_VSP*( a1*sin(b1*alpha+c1) + ...
                a2*sin(b2*alpha+c2) + ...
                a3*sin(b3*alpha+c3) + ...
                a4*sin(b4*alpha+c4) + ...
                a5*sin(b5*alpha+c5) + ...
                a6*sin(b6*alpha+c6));

== matlab function NowWereHere2018/Controller/CtrlCustom_SLX/Controller/Controller ==
  data: eta input; etaDot input; tau output; mode input; StartPos input; endPos input; sDot input; sDotDot input; s input; sDotNew output
function [tau,sDotNew] = fcn(eta,etaDot,mode,StartPos,endPos,sDot,sDotDot,s) %s should be the final input for aestetic reasons
%tuning parameters:
if mode==1 %straight line
    %tuning
    mu=1; %mu>0
    KpVec=[1,1,1];
    Kp=diag(KpVec);
    K2=diag([1,1,1]);
    
    
    %Path Parametrisation
    etaD=zeros(3,1);
    etaDs=zeros(3,1);
    etaDss = [0;0;0];
    Trajectory = (endPos(:,1) - StartPos(:,1))*s + StartPos(:,1);
    DesiredHeading = atan((endPos(2)-StartPos(2))/(endPos(1)-StartPos(1)));
    etaD(1)= Trajectory(1);
    etaD(2)= Trajectory(2);
    etaD(3)= DesiredHeading;
    %HeadingS = 0;
    %HeadingSS = 0;
    etaDs(1) = (endPos(1) - StartPos(1));
    etaDs(2) = (endPos(2) - StartPos(2));
    xds=etaDs(1);
    yds=etaDs(2);
    xdss=0;
    ydss=0;
    
else %ellipsoid
    %tuning
    mu=1; %mu>0, mu<0.1
    KpVec=[1,1,1];
    Kp=diag([1,1,1]);
    K2=diag([1,1,1]);
    %calculation
    etaD = zeros(3,1);
    Trajectory=zeros(3,1);
    etaDs = zeros(3,1);
    etaDss = zeros(3,1);

    c_x = (endPos(1)-StartPos(1))/2;
    c_y = (endPos(2)-StartPos(2))/2;
    r_x = sqrt(c_x^2 + c_y^2);
    r_y = 1/4 * r_x;
    Trajectory(1) = r_x*cos(2*pi*s);
    Trajectory(2) = r_y*sin(2*pi*s);
    DesiredHeading = atan((r_y*sin(2*pi*s)+c_y)/(r_x*cos(2*pi*s)+c_x));
    etaDs(1) = -2*pi*r_x*sin(2*pi*s);
    etaDs(2) = 2*pi*r_y*cos(2*pi*s);
    etaDs(3) = ((-2*pi*r_x*sin(2*pi*s))*(-4*pi^2*r_y*sin(2*pi*s)) - ...
    (-4*pi^2*r_x*cos(2*pi*s)*-2*pi*r_y*cos(2*pi*s))) /...
    ((-2*pi*r_x*sin(2*pi*s))^2 + (2*pi*r_y*cos(2*pi*s))^2);
    
    etaDss(1) = -4*pi^2*cos(2*pi*s);
    
    etaDss(2) = -4*pi^2*sin(2*pi*s);
    
    etaDss(3) = 2*((-2*pi*r_x*sin(2*pi*s))*(-4*pi^2*r_y*sin(2*pi*s)) - ...
    (-4*pi^2*r_x*cos(2*pi*s)*-2*pi*r_y*cos(2*pi*s)))* ...
    (-2*pi*r_x*sin(2*pi*s)*-4*pi^2*r_x*cos(2*pi*s) + ...
    2*pi*r_y*cos(2*pi*s)*-4*pi^2*r_y*sin(2*pi*s)) /...
    ((-2*pi*r_x*sin(2*pi*s))^2 + (2*pi*r_y*cos(2*pi*s))^2)^2;
    etaD(1,1)= Trajectory(1);
    etaD(2,1)= Trajectory(2);
    etaD(3,1)= DesiredHeading;
    
    xds=etaDs(1);
    yds=etaDs(2);
    xdss=etaDss(1);
    ydss=etaDss(2);
end




%constants
R=[cos(eta(3,1)),-sin(eta(3,1)),0;sin(eta(3,1)),cos(eta(3,1)),0;0,0,1];
Rt=transpose(R);
M=[16,0,0;0,24,0.53;0,0.53,2.8];
D=[0.66,0,0;0,1.3,2.8;0,0,1.9];
Us=sDot*sqrt(xds^2+yds^2);
nu=R*etaDot;

Uss=sDotDot*sqrt(xds^2+yds^2)+((sDot*(xds*xdss+yds*ydss)/(sqrt(xds^2+yds^2))));

%actual controller eqs

z1=Rt*(eta-etaD);
alpha1=-Kp*z1+Rt*etaDs*Us;
alpha1s=Rt*(etaDss*Us+etaDs*Uss);
sigma1=-KpVec*Rt; %should Rt be derivated here?

V1s=-transpose(z1)*Rt*etaDs;


z2=nu+alpha1;


tau=-z1+D*nu+M*alpha1s*Us+M*sigma1'-K2*z2;
sDotNew=(Us-(mu/norm(etaDs))*V1s)';
end
